simulink library "enginelib"  (Simulink 6.6)
libraries: enginelib x2, engine_AMT180_lib x1, engine_AMT280_lib x1, engine_T2_lib x1, engine_JetCatP120SE_lib x1, engine_JetCatP70_lib x1, engine_S2_lib x1, simulink x1
settings Model: Creator=cox  LastModifiedBy=amurch  ExtModeAutoUpdateStatusClock=off

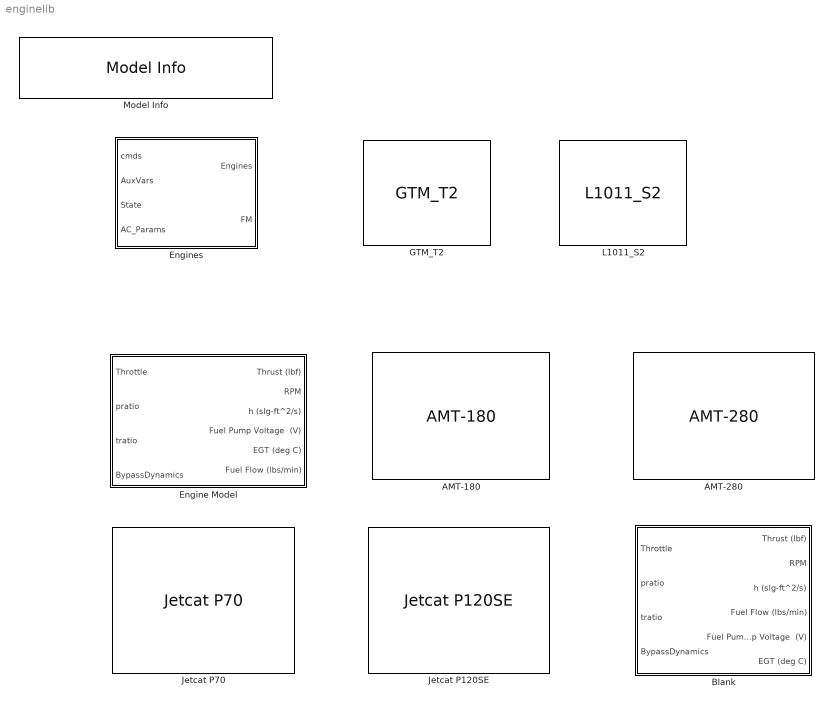
== system enginelib ==
  AMT-180 : engine_AMT180_lib/AMT-180  SystemSampleTime=-1
  AMT-280 : engine_AMT280_lib/AMT-280  SystemSampleTime=-1
  Blank : Subsystem
      mask init:
      | % Curve fit parameters for AMT-280 Model
      | Coeff_thrust   = [ 5.7372e-05  -5.2629e-03   3.1586e-01  -5.1517e+00];
      | Coeff_throttle = [ -4.3078e-03   1.1110e+00   2.9012e+01];
      | Coeff_fuelflow = [ 1.0140e-04  -1.5867e-03   2.0125e-01];
      | Coeff_tau      = [ -2.2400e-02   2.9948e+00];
      | 
      | 
      | % Equvalent Shaft parameters for engine
      | shaft_dia = 0.75/12.0;       % diameter of rotating turbine in feet 
      | shaft_len = 6.25/12.0;       % length of rotating turbine in feet   
      | density   = 15.2;            % mass density of steel in slugs/ft^3
  Engine Model : Subsystem  BlockChoice=Blank
      settings: TemplateBlock=self  MemberBlocks=AMT-180,AMT-280,Blank,Jetcat P120SE,Jetcat P70
  Engines : Subsystem  BlockChoice=L1011_S2
      settings: TemplateBlock=self  MemberBlocks=GTM_T2,L1011_S2
  GTM_T2 : engine_T2_lib/GTM_T2  SystemSampleTime=-1
  Jetcat P120SE : engine_JetCatP120SE_lib/Jetcat P120SE  SystemSampleTime=-1
  Jetcat P70 : engine_JetCatP70_lib/Jetcat P70  SystemSampleTime=-1
  L1011_S2 : engine_S2_lib/L1011_S2  SystemSampleTime=-1
  Model Info : simulink/Model-Wide Utilities/Model Info  SystemSampleTime=-1  InitialBlockCM=none  BlockCM=none  Frame=on  DisplayStringWithTags=|  HorizontalTextAlignment=Center  LeftAlignmentValue=0.5  SourceBlockDiagram=enginelib  TagMaxNumber=20
      | engine library
      | 
      | Model Version: %<ModelVersion>
      | Last modifed by %<LastModifiedBy> on %<LastModificationDate>

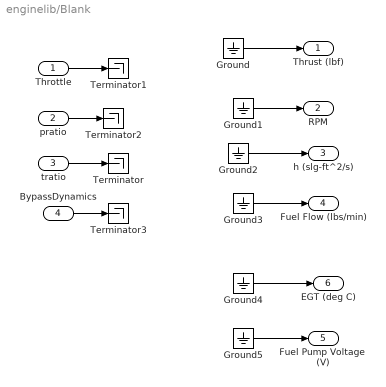
== system enginelib/Blank ==
  Throttle : Inport
  pratio : Inport  Port=2
  tratio : Inport  Port=3
  BypassDynamics : Inport  Port=4
  Ground{,1..5} (6 alike) : Ground
  Terminator{,1..3} (4 alike) : Terminator
  Thrust (lbf) : Outport
  RPM : Outport  Port=2
  h (slg-ft^2/s) : Outport  Port=3
  Fuel Flow (lbs/min) : Outport  Port=4
  Fuel Pump Voltage  (V) : Outport  Port=5
  EGT (deg C) : Outport  Port=6
  wires:
  Throttle/1 -> Terminator1/1
  pratio/1 -> Terminator2/1
  tratio/1 -> Terminator/1
  Ground/1 -> Thrust (lbf)/1
  Ground1/1 -> RPM/1
  Ground2/1 -> h (slg-ft^2/s)/1
  Ground5/1 -> Fuel Pump Voltage  (V)/1
  Ground4/1 -> EGT (deg C)/1
  Ground3/1 -> Fuel Flow (lbs/min)/1
  BypassDynamics/1 -> Terminator3/1

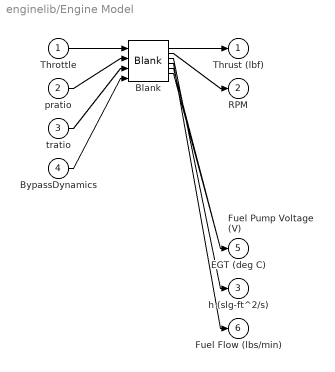
== system enginelib/Engine Model ==
  Throttle : Inport
  pratio : Inport  Port=2
  tratio : Inport  Port=3
  BypassDynamics : Inport  Port=4
  Blank : enginelib/Blank  SystemSampleTime=-1
  Thrust (lbf) : Outport
  RPM : Outport  Port=2
  h (slg-ft^2/s) : Outport  Port=3
  Fuel Pump Voltage  (V) : Outport  Port=4
  EGT (deg C) : Outport  Port=5
  Fuel Flow (lbs/min) : Outport  Port=6
  wires:
  Throttle/1 -> Blank/1
  pratio/1 -> Blank/2
  tratio/1 -> Blank/3
  BypassDynamics/1 -> Blank/4
  Blank/1 -> Thrust (lbf)/1
  Blank/2 -> RPM/1
  Blank/3 -> h (slg-ft^2/s)/1
  Blank/4 -> Fuel Flow (lbs/min)/1
  Blank/5 -> Fuel Pump Voltage  (V)/1
  Blank/6 -> EGT (deg C)/1

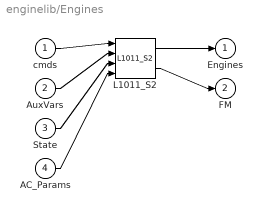
== system enginelib/Engines ==
  cmds : Inport
  AuxVars : Inport  Port=2
  State : Inport  Port=3
  AC_Params : Inport  Port=4
  L1011_S2 : enginelib/L1011_S2  SystemSampleTime=-1
  Engines : Outport
  FM : Outport  Port=2
  wires:
  cmds/1 -> L1011_S2/1
  AuxVars/1 -> L1011_S2/2
  State/1 -> L1011_S2/3
  AC_Params/1 -> L1011_S2/4
  L1011_S2/1 -> Engines/1
  L1011_S2/2 -> FM/1
